simulink library "INT_EngReq_SmkLimCalc"  (R2016b)
settings: Solver=VariableStepAuto  StartTime=0.0  StopTime=10.0  RelTol=1e-3
settings Model: Creator=bianxuyin  LastModifiedBy=bianxuyin

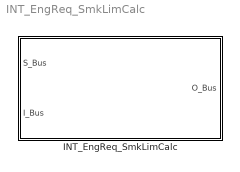
== system INT_EngReq_SmkLimCalc ==
  INT_EngReq_SmkLimCalc : Subsystem

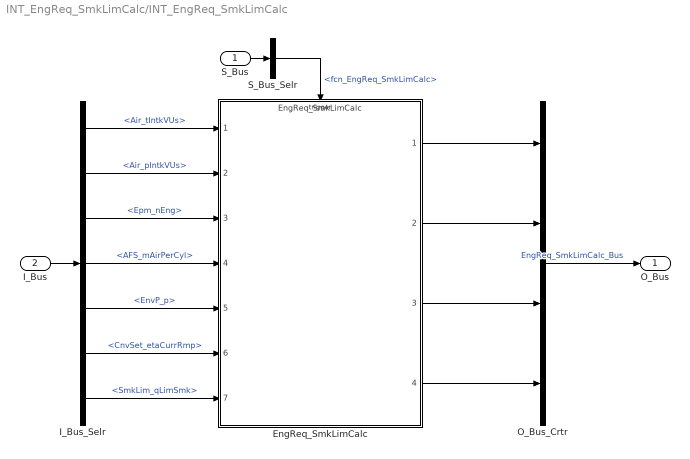
== system INT_EngReq_SmkLimCalc/INT_EngReq_SmkLimCalc ==
  S_Bus : Inport
  I_Bus : Inport  Port=2
  EngReq_SmkLimCalc : ModelReference  ModelNameDialog=EngReq_SmkLimCalc  SimulationMode=Normal  ModelReferenceVersion=1.31  TriggerPortName=function  TriggerPortTriggerType=function-call  TriggerPortStatesWhenEnabling=held
  I_Bus_Selr : BusSelector  OutputSignals=Air_tIntkVUs,Air_pIntkVUs,Epm_nEng,AFS_mAirPerCyl,EnvP_p,CnvSet_etaCurrRmp,SmkLim_qLimSmk
  O_Bus_Crtr : BusCreator  Inputs=4
  S_Bus_Selr : BusSelector  OutputSignals=fcn_EngReq_SmkLimCalc
  O_Bus : Outport
  wires:
  S_Bus_Selr/1 -> EngReq_SmkLimCalc/Trigger  "<fcn_EngReq_SmkLimCalc>"
  S_Bus/1 -> S_Bus_Selr/1
  I_Bus/1 -> I_Bus_Selr/1
  I_Bus_Selr/1 -> EngReq_SmkLimCalc/1  "<Air_tIntkVUs>"
  I_Bus_Selr/2 -> EngReq_SmkLimCalc/2  "<Air_pIntkVUs>"
  I_Bus_Selr/3 -> EngReq_SmkLimCalc/3  "<Epm_nEng>"
  I_Bus_Selr/4 -> EngReq_SmkLimCalc/4  "<AFS_mAirPerCyl>"
  I_Bus_Selr/5 -> EngReq_SmkLimCalc/5  "<EnvP_p>"
  I_Bus_Selr/6 -> EngReq_SmkLimCalc/6  "<CnvSet_etaCurrRmp>"
  I_Bus_Selr/7 -> EngReq_SmkLimCalc/7  "<SmkLim_qLimSmk>"
  O_Bus_Crtr/1 -> O_Bus/1  "EngReq_SmkLimCalc_Bus"
  EngReq_SmkLimCalc/1 -> O_Bus_Crtr/1
  EngReq_SmkLimCalc/2 -> O_Bus_Crtr/2
  EngReq_SmkLimCalc/3 -> O_Bus_Crtr/3
  EngReq_SmkLimCalc/4 -> O_Bus_Crtr/4
